simulink model "damper_pid"  (R2019b)
settings: Solver=VariableStepAuto  StartTime=0.0  StopTime=sim_time  RelTol=1e-3
values from neighbouring files (symbols this model uses):
  b = 50    [adaptive_cruise.m]    (also in damper_pid_run.m = 10; dc_motor_run.m = 3.5077e-06; pid_tune_run.m = 10; spring_damp.m = 0.5)
  k = 20    [damper_pid_run.m]    (also in pid_tune_run.m; spring_damp.m)
  Kd = 50    [damper_pid_run.m]    (also in pid_tune_run.m = 2.438)
  Ki = 40    [adaptive_cruise.m]    (also in damper_pid_run.m = 300; pid_tune_run.m = 114.7)
  Kp = 800    [adaptive_cruise.m]    (also in damper_pid_run.m = 350; pid_tune_run.m = 37.8)
  M = 1    [damper_pid_run.m]    (also in pid_tune_run.m; spring_damp.m)
  step_value = 1    [damper_pid_run.m]
settings Model: Creator=dgander  LastModifiedBy=dgander

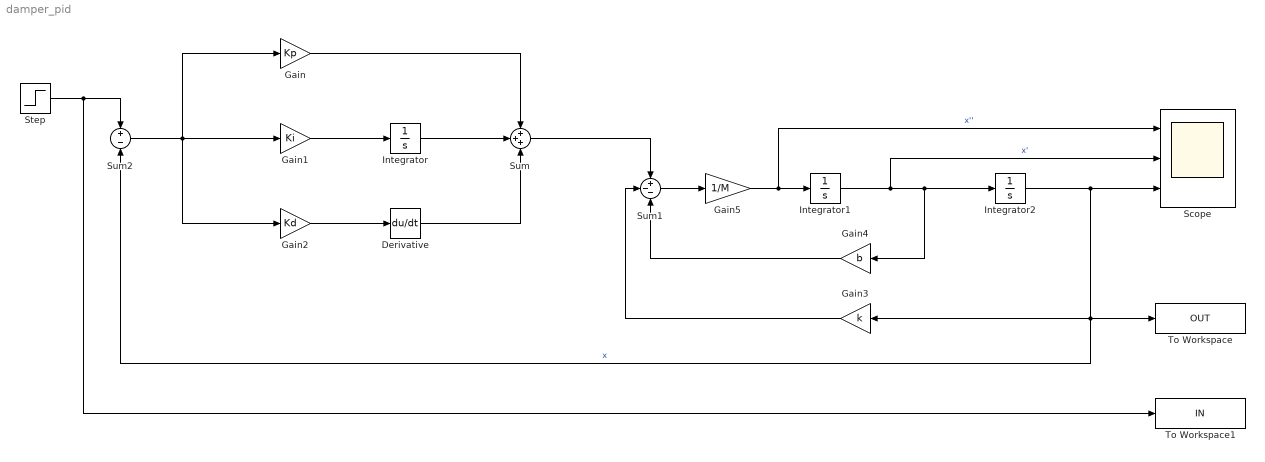
== system damper_pid ==
  Derivative : Derivative
  Gain : Gain  Gain=Kp
  Gain1 : Gain  Gain=Ki
  Gain2 : Gain  Gain=Kd
  Gain3 : Gain  Gain=k
  Gain4 : Gain  Gain=b
  Gain5 : Gain  Gain=1/M
  Integrator : Integrator
  Integrator1 : Integrator
  Integrator2 : Integrator
  Scope : Scope  NumInputPorts=3
  Step : Step  After=step_value  SampleTime=0
  Sum : Sum  Inputs=+++
  Sum1 : Sum  Inputs=+--
  Sum2 : Sum  Inputs=+-
  To Workspace : ToWorkspace  VariableName=OUT  SaveFormat=Timeseries  SampleTime=-1
  To Workspace1 : ToWorkspace  VariableName=IN  SaveFormat=Timeseries  SampleTime=-1
  wires:
  Sum/1 -> Sum1/1
  Sum2/1 -> Gain2/1, Gain1/1, Gain/1
  Gain2/1 -> Derivative/1
  Derivative/1 -> Sum/3
  Gain1/1 -> Integrator/1
  Integrator/1 -> Sum/2
  Gain/1 -> Sum/1
  Sum1/1 -> Gain5/1
  Gain3/1 -> Sum1/2
  Gain4/1 -> Sum1/3
  Integrator2/1 -> To Workspace/1, Sum2/2, Gain3/1, Scope/3  "x"
  Integrator1/1 -> Scope/2, Gain4/1, Integrator2/1  "x'"
  Gain5/1 -> Scope/1, Integrator1/1  "x''"
  Step/1 -> Sum2/1, To Workspace1/1
